simulink model "relayFeedback"  (R2019a)
settings: Solver=VariableStepAuto  StartTime=0.0  StopTime=50  RelTol=1e-3
settings Model: Creator=Administrator  LastModifiedBy=Administrator

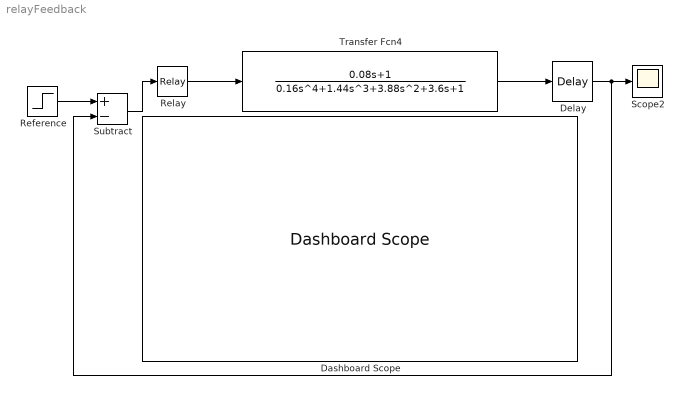
== system relayFeedback ==
  Dashboard Scope : DashboardScope
  Delay : TransportDelay  DelayTime=3
  Reference : Step  After=0  SampleTime=0
  Relay : Relay  OnOutputValue=0.01  OffOutputValue=-0.01
  Scope2 : Scope
  Subtract : Sum  Inputs=+-
  Transfer Fcn4 : TransferFcn  Numerator=[0.08 1]  Denominator=[0.16 1.44 3.88 3.6 1]
  wires:
  Delay/1 -> Subtract/2, Scope2/1
  Subtract/1 -> Relay/1
  Reference/1 -> Subtract/1
  Relay/1 -> Transfer Fcn4/1
  Transfer Fcn4/1 -> Delay/1
